simulink model "ex1sim"  (R2015a)
settings: Solver=ode45  StartTime=0.0  StopTime=10.0  RelTol=1e-3
values from neighbouring files (symbols this model uses):
  Ts = 1    [ex1.m]    (also in ex2.m = 0.5; ex4.m = 0.05)
settings Model: Creator=BPeixoto  LastModifiedBy=BPeixoto

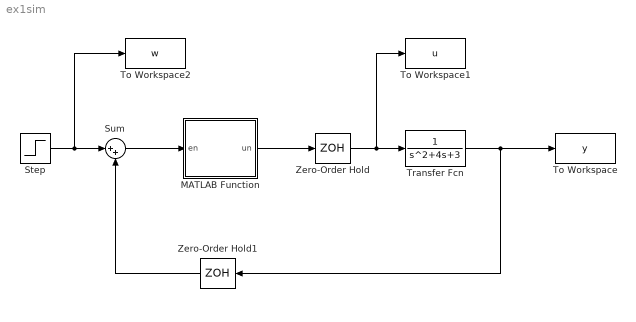
== system ex1sim ==
  MATLAB Function : MATLAB Function  TreatAsAtomicUnit=on
  Step : Step  SampleTime=Ts
  Sum : Sum  Inputs=|++
  To Workspace : ToWorkspace  VariableName=y  SaveFormat=Timeseries  SampleTime=Ts
  To Workspace1 : ToWorkspace  VariableName=u  SaveFormat=Timeseries  SampleTime=Ts
  To Workspace2 : ToWorkspace  VariableName=w  SaveFormat=Timeseries  SampleTime=Ts
  Transfer Fcn : TransferFcn  Denominator=[1 4 3]
  Zero-Order Hold : ZeroOrderHold  SampleTime=Ts
  Zero-Order Hold1 : ZeroOrderHold  SampleTime=Ts
  wires:
  Zero-Order Hold1/1 -> Sum/2
  MATLAB Function/1(un) -> Zero-Order Hold/1
  Sum/1 -> MATLAB Function/1(en)
  Zero-Order Hold/1 -> To Workspace1/1, Transfer Fcn/1
  Transfer Fcn/1 -> To Workspace/1, Zero-Order Hold1/1
  Step/1 -> To Workspace2/1, Sum/1

== matlab function ex1sim/MATLAB Function ==
  data: un output; en input; params parameter
function un = fcn(en, params)
    persistent un_1;
    persistent en_1;
    
    if(isempty(un_1))
        un_1 = 0;
    end
    
    if(isempty(en_1))
        en_1 = 0;
    end
    
    a1 = params.a1;
    a0 = params.a0;
    b1 = params.b1;
    b0 = params.b0;
    
    un = (b1/a0)*en_1 + (b0/a0)*en - (a1/a0)*en;
    
    un_1 = un;
    en_1 = en;
